simulink model "s_as_lqr"  (Simulink 8.7)
settings: Solver=ode1  StartTime=0.0  StopTime=inf  FixedStep=0.001  RelTol=1e-3
values from neighbouring files (symbols this model uses):
  A = [ 0 1 0 -1 ... (first row only)    [FitnessFunc.m]    (also in FitnessFunc_ISE.m; FitnessFunc_ITAE.m; setup_as.m)
  B = [0  0 ... (first row only)    [FitnessFunc.m]    (also in FitnessFunc_ISE.m; FitnessFunc_ITAE.m; setup_as.m = [0  0 ; 0 1/ms ; -1  0 ; bus/mu -1/mu ])
  C = [ 1 0 0 0 ... (first row only)    [FitnessFunc.m]    (also in FitnessFunc_ISE.m; FitnessFunc_ITAE.m; setup_as.m = [ 1 0 0 0 ; -ks/ms -bs/ms 0 bs/ms ])
  D = [0 0 ... (first row only)    [FitnessFunc.m]    (also in FitnessFunc_ISE.m; FitnessFunc_ITAE.m; setup_as.m = zeros(6,2); D(6,2)=1/ms)
  K = lqr( A, B(:,2), Q, R )    [setup_as.m]
libraries: simulink x8, quarc_library x1
settings Model: Creator=DCrymble  LastModifiedBy=amolki  SimulationMode=external  ExtModeTrigDuration=50000
settings SolverCC: PositivePriorityOrder=on
settings DataIOCC: SignalLoggingSaveFormat=ModelDataLogs
settings OptimizationCC: BooleanDataType=off  OptimizeBlockIOStorage=off  BufferReuse=off  GlobalBufferReuse=off  ExpressionFolding=off  ExpressionDepthLimit=2147483647  LocalBlockOutputs=off  InitFltsAndDblsToZero=on
settings DebuggingCC: SolverPrmCheckMsg=warning  FcnCallInpInsideContextMsg=UseLocalSettings  StateNameClashWarn=warning  StrictBusMsg=Warning
settings SFSimCC: SimParseCustomCode=off
settings RTWCC: SystemTargetFile=quarc_windows.tlc  TemplateMakefile=quarc_default_tmf  Description=QuaRC Win32 Target
settings STFCustomTargetCC: TargetPreCompLibLocation=C:\PROGRA~2\QUARC\lib\2012b\windows\release  GeneratePreprocessorConditionals=Disable all  CPPClassGenCompliant=on  SystemTargetFile=quarc_windows.tlc
settings GRTTargetCC: TargetPreCompLibLocation=C:\PROGRA~3\QUARC\lib\2016a\windows\release  ParMdlRefBuildCompliant=off  CompOptLevelCompliant=off  ConcurrentExecutionCompliant=off  CombineOutputUpdateFcns=off  MatFileLogging=off  GRTInterface=on  UseToolchainInfoCompliant=off  ExtMode=on  ExtModeMexFile=quarc_comm

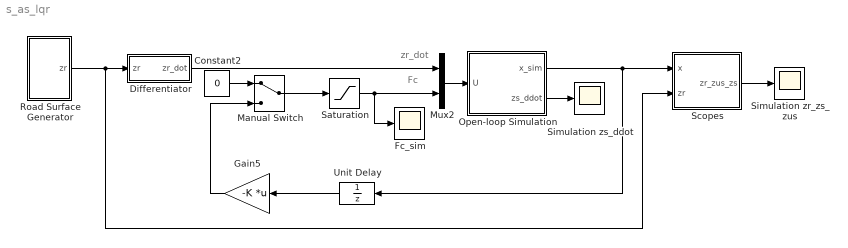
== system s_as_lqr ==
  note: zr_dot
  note: Fc
  Constant2 : Constant  Value=0
  Differentiator : Subsystem
  Fc_sim : Scope
  Gain5 : Gain  Gain=-K  Multiplication=Matrix(K*u)
  Manual Switch : ManualSwitch
  Mux2 : Mux  Inputs=2
  Open-loop Simulation : Subsystem
  Road Surface Generator : Subsystem
  Saturation : Saturate  UpperLimit=38.3  LowerLimit=-38.3
  Scopes : Subsystem
  Simulation zr_zs_zus : Scope
  Simulation zs_ddot : Scope
  Unit Delay : UnitDelay  SampleTime=-1
  wires:
  Differentiator/1(zr_dot) -> Mux2/1
  Constant2/1 -> Manual Switch/1
  Manual Switch/1 -> Saturation/1
  Mux2/1 -> Open-loop Simulation/1(U)
  Scopes/1(zr_zus_zs) -> Simulation zr_zs_zus/1
  Saturation/1 -> Mux2/2, Fc_sim/1
  Gain5/1 -> Manual Switch/2
  Open-loop Simulation/1(x_sim) -> Unit Delay/1, Scopes/1(x)
  Unit Delay/1 -> Gain5/1
  Road Surface Generator/1(zr) -> Scopes/2(zr), Differentiator/1(zr)
  Open-loop Simulation/2(zs_ddot) -> Simulation zs_ddot/1

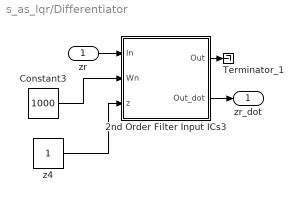
== system s_as_lqr/Differentiator ==
  zr : Inport
  2nd Order Filter Input ICs3 : Subsystem
  Constant3 : Constant  Value=1000
  Terminator_1 : Terminator
  z4 : Constant
  zr_dot : Outport
  wires:
  Constant3/1 -> 2nd Order Filter Input ICs3/2(Wn)
  z4/1 -> 2nd Order Filter Input ICs3/3(z)
  zr/1 -> 2nd Order Filter Input ICs3/1(In)
  2nd Order Filter Input ICs3/2(Out_dot) -> zr_dot/1
  2nd Order Filter Input ICs3/1(Out) -> Terminator_1/1

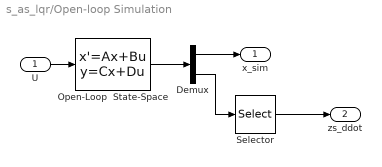
== system s_as_lqr/Open-loop Simulation ==
  U : Inport
  Demux : Demux  Outputs=[4 2]
  Open-Loop  State-Space : StateSpace  A=A  B=B  C=cat(1,eye(4), C)  D=D  X0=0
  Selector : Selector  InputPortWidth=2  IndexOptions=Index vector (dialog)  Indices=[2]  OutputSizes=1
  x_sim : Outport
  zs_ddot : Outport  Port=2
  wires:
  Open-Loop  State-Space/1 -> Demux/1
  Demux/1 -> x_sim/1
  U/1 -> Open-Loop  State-Space/1
  Demux/2 -> Selector/1
  Selector/1 -> zs_ddot/1

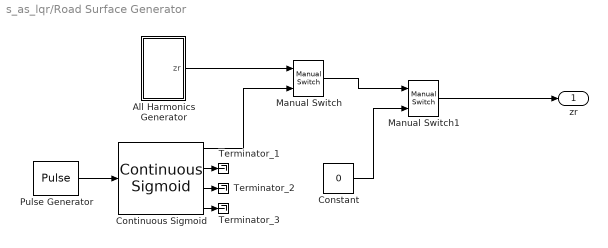
== system s_as_lqr/Road Surface Generator ==
  All Harmonics Generator : Subsystem
  Constant : Constant  Value=0
  Continuous Sigmoid : quarc_library/Sources/Sigmoids/Continuous Sigmoid  params_source=Internal (dialog parameters)  max_velocity=.6/3  max_acceleration=20  initial_position=0  initial_velocity=0  hold_off=0.5  input_sample_time=-1  output_sample_time=qc_get_step_size
  Manual Switch : simulink/Signal Routing/Manual Switch  sw=0  action=0  varsize=off
  Manual Switch1 : simulink/Signal Routing/Manual Switch  sw=1  action=0  varsize=off
  Pulse Generator : DiscretePulseGenerator  PulseType=Time based  Amplitude=0.02  Period=3  PulseWidth=50  PhaseDelay=.1
  Terminator_1 : Terminator
  Terminator_2 : Terminator
  Terminator_3 : Terminator
  zr : Outport
  wires:
  Pulse Generator/1 -> Continuous Sigmoid/1
  All Harmonics Generator/1(zr) -> Manual Switch/1
  Continuous Sigmoid/1 -> Manual Switch/2
  Constant/1 -> Manual Switch1/2
  Manual Switch/1 -> Manual Switch1/1
  Continuous Sigmoid/2 -> Terminator_1/1
  Continuous Sigmoid/3 -> Terminator_2/1
  Continuous Sigmoid/4 -> Terminator_3/1
  Manual Switch1/1 -> zr/1

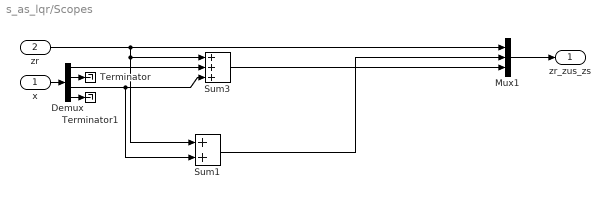
== system s_as_lqr/Scopes ==
  x : Inport
  zr : Inport  Port=2
  Demux : Demux
  Mux1 : Mux  Inputs=3
  Sum1 : Sum  Inputs=2  SaturateOnIntegerOverflow=on  InputSameDT=on  OutDataTypeStr=Inherit: Same as first input
  Sum3 : Sum  Inputs=3  SaturateOnIntegerOverflow=on  InputSameDT=on  OutDataTypeStr=Inherit: Same as first input
  Terminator : Terminator
  Terminator1 : Terminator
  zr_zus_zs : Outport
  wires:
  Demux/1 -> Sum3/2
  Demux/3 -> Sum3/3, Sum1/2
  zr/1 -> Mux1/1, Sum3/1, Sum1/1
  x/1 -> Demux/1
  Sum1/1 -> Mux1/2
  Sum3/1 -> Mux1/3
  Mux1/1 -> zr_zus_zs/1
  Demux/2 -> Terminator/1
  Demux/4 -> Terminator1/1

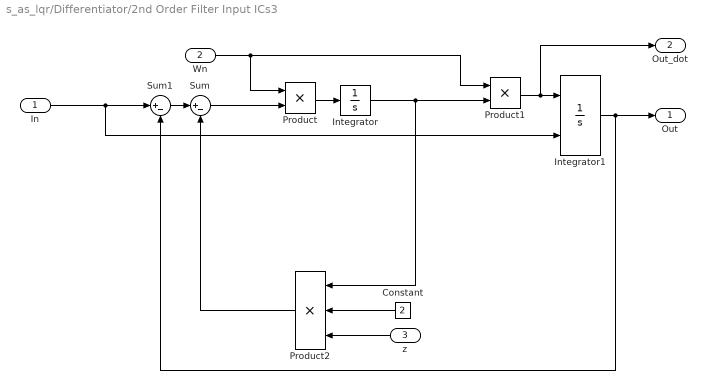
== system s_as_lqr/Differentiator/2nd Order Filter Input ICs3 ==
  In : Inport
  Wn : Inport  Port=2
  z : Inport  Port=3
  Constant : Constant  Value=2
  Integrator : Integrator
  Integrator1 : Integrator  InitialConditionSource=external
  Product : Product  RndMeth=Zero
  Product1 : Product  RndMeth=Zero
  Product2 : Product  Inputs=3  RndMeth=Zero
  Sum : Sum  Inputs=|+-
  Sum1 : Sum  Inputs=|+-
  Out : Outport
  Out_dot : Outport  Port=2
  wires:
  Constant/1 -> Product2/2
  z/1 -> Product2/3
  Product2/1 -> Sum/2
  In/1 -> Integrator1/2, Sum1/1
  Sum1/1 -> Sum/1
  Integrator1/1 -> Out/1, Sum1/2
  Integrator/1 -> Product2/1, Product1/2
  Product1/1 -> Out_dot/1, Integrator1/1
  Wn/1 -> Product1/1, Product/1
  Sum/1 -> Product/2
  Product/1 -> Integrator/1

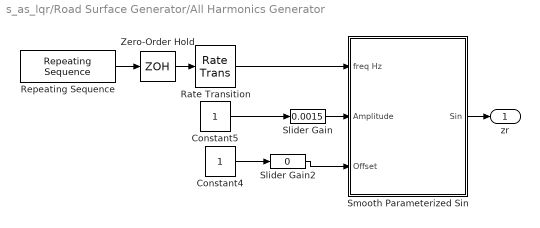
== system s_as_lqr/Road Surface Generator/All Harmonics Generator ==
  Constant4 : Constant
  Constant5 : Constant
  Rate Transition : RateTransition
  Repeating Sequence : simulink/Sources/Repeating Sequence  rep_seq_t=[0 30 30.1 ]  rep_seq_y=[1 8 1 ]
  Slider Gain : simulink/Math Operations/Slider Gain  low=0  gain=0.0015  high=0.002
  Slider Gain2 : simulink/Math Operations/Slider Gain  low=-10  gain=0  high=10
  Smooth Parameterized Sin : Subsystem  mask(Smooth Parameterized Sin Wave){}
      mask help:
      | Sin wave that will smoothly and continuously change as input
      | parameters are changed.
      |
      | Out = Amplitude * sin(freq*t) +offset
  Zero-Order Hold : ZeroOrderHold  SampleTime=.1
  zr : Outport
  wires:
  Slider Gain/1 -> Smooth Parameterized Sin/2(Amplitude)
  Slider Gain2/1 -> Smooth Parameterized Sin/3(Offset)
  Constant4/1 -> Slider Gain2/1
  Constant5/1 -> Slider Gain/1
  Repeating Sequence/1 -> Zero-Order Hold/1
  Zero-Order Hold/1 -> Rate Transition/1
  Rate Transition/1 -> Smooth Parameterized Sin/1(freq Hz)
  Smooth Parameterized Sin/1(Sin) -> zr/1

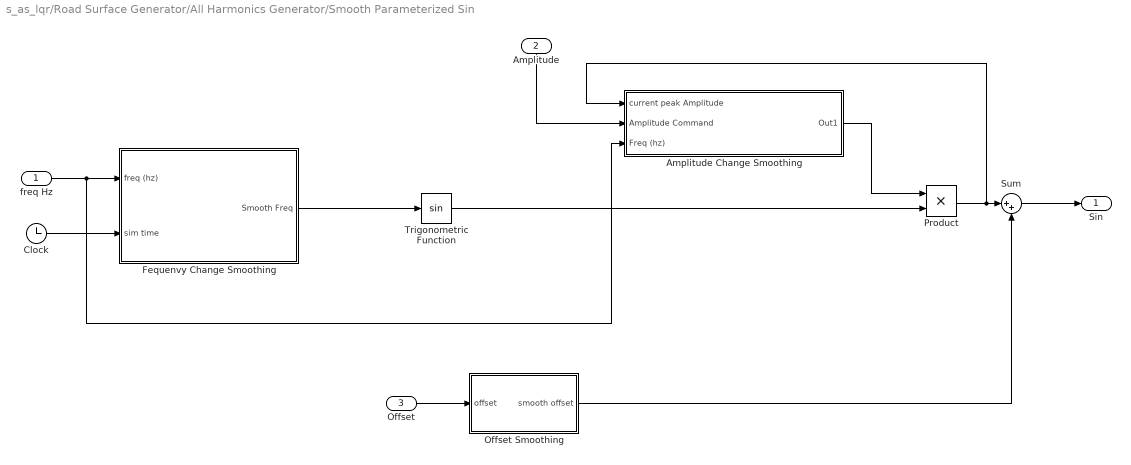
== system s_as_lqr/Road Surface Generator/All Harmonics Generator/Smooth Parameterized Sin ==
  freq Hz : Inport
  Amplitude : Inport  Port=2
  Offset : Inport  Port=3
  Amplitude Change Smoothing : Subsystem
  Clock : Clock
  Fequenvy Change Smoothing : Subsystem
  Offset Smoothing : Subsystem
  Product : Product  RndMeth=Zero
  Sum : Sum  Inputs=|++
  Trigonometric Function : Trigonometry
  Sin : Outport
  wires:
  Sum/1 -> Sin/1
  Clock/1 -> Fequenvy Change Smoothing/2(sim time)
  freq Hz/1 -> Fequenvy Change Smoothing/1(freq (hz)), Amplitude Change Smoothing/3(Freq (hz))
  Fequenvy Change Smoothing/1(Smooth Freq) -> Trigonometric Function/1
  Trigonometric Function/1 -> Product/2
  Offset Smoothing/1(smooth offset) -> Sum/2
  Offset/1 -> Offset Smoothing/1(offset)
  Product/1 -> Sum/1, Amplitude Change Smoothing/1(current peak Amplitude)
  Amplitude Change Smoothing/1(Out1) -> Product/1
  Amplitude/1 -> Amplitude Change Smoothing/2(Amplitude Command)

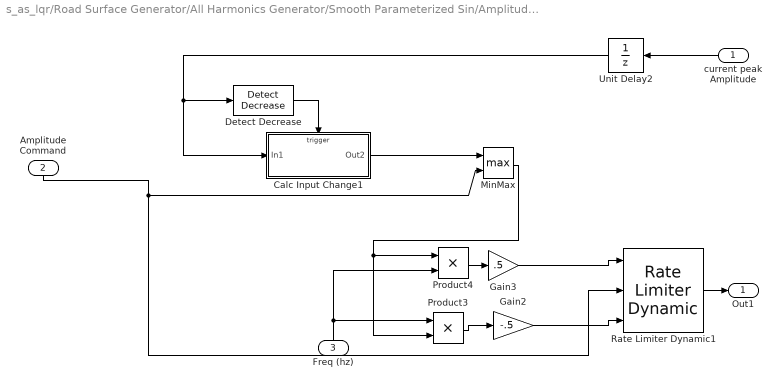
== system s_as_lqr/Road Surface Generator/All Harmonics Generator/Smooth Parameterized Sin/Amplitude Change Smoothing ==
  current peak Amplitude : Inport
  Amplitude Command : Inport  Port=2
  Freq (hz) : Inport  Port=3
  Calc Input Change1 : Subsystem  TreatAsAtomicUnit=on
  Detect Decrease : simulink/Logic and Bit Operations/Detect Decrease  vinit=0.0  InputProcessing=Inherited  OutDataTypeStr=uint8
  Gain2 : Gain  Gain=-.5
  Gain3 : Gain  Gain=.5
  MinMax : MinMax  Function=max  Inputs=2
  Product3 : Product  RndMeth=Zero
  Product4 : Product  RndMeth=Zero
  Rate Limiter Dynamic1 : simulink/Discontinuities/Rate Limiter Dynamic
  Unit Delay2 : UnitDelay  SampleTime=-1
  Out1 : Outport
  wires:
  Gain2/1 -> Rate Limiter Dynamic1/3
  Gain3/1 -> Rate Limiter Dynamic1/1
  Amplitude Command/1 -> MinMax/2, Rate Limiter Dynamic1/2
  Product3/1 -> Gain2/1
  Product4/1 -> Gain3/1
  Detect Decrease/1 -> Calc Input Change1/Trigger
  Calc Input Change1/1(Out2) -> MinMax/1
  Unit Delay2/1 -> Calc Input Change1/1(In1), Detect Decrease/1
  MinMax/1 -> Product4/1, Product3/2
  current peak Amplitude/1 -> Unit Delay2/1
  Freq (hz)/1 -> Product3/1, Product4/2
  Rate Limiter Dynamic1/1 -> Out1/1

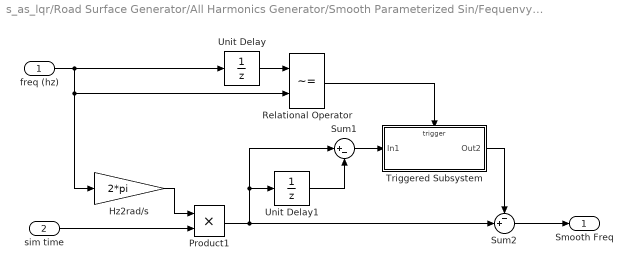
== system s_as_lqr/Road Surface Generator/All Harmonics Generator/Smooth Parameterized Sin/Fequenvy Change Smoothing ==
  freq (hz) : Inport
  sim time : Inport  Port=2
  Hz2rad/s : Gain  Gain=2*pi
  Product1 : Product  RndMeth=Zero
  Relational Operator : RelationalOperator  Operator=~=  OutDataTypeStr=boolean
  Sum1 : Sum  Inputs=|+-
  Sum2 : Sum  Inputs=-+|
  Triggered Subsystem : Subsystem  TreatAsAtomicUnit=on
  Unit Delay : UnitDelay  SampleTime=-1
  Unit Delay1 : UnitDelay  SampleTime=-1
  Smooth Freq : Outport
  wires:
  Triggered Subsystem/1(Out2) -> Sum2/1
  Unit Delay1/1 -> Sum1/2
  Relational Operator/1 -> Triggered Subsystem/Trigger
  Sum1/1 -> Triggered Subsystem/1(In1)
  Unit Delay/1 -> Relational Operator/1
  Product1/1 -> Sum2/2, Sum1/1, Unit Delay1/1
  freq (hz)/1 -> Unit Delay/1, Relational Operator/2, Hz2rad/s/1
  Sum2/1 -> Smooth Freq/1
  sim time/1 -> Product1/2
  Hz2rad/s/1 -> Product1/1

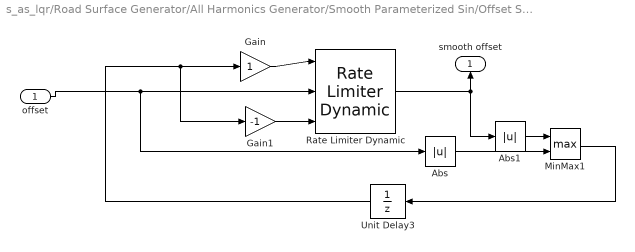
== system s_as_lqr/Road Surface Generator/All Harmonics Generator/Smooth Parameterized Sin/Offset Smoothing ==
  offset : Inport
  Abs : Abs
  Abs1 : Abs
  Gain : Gain
  Gain1 : Gain  Gain=-1
  MinMax1 : MinMax  Function=max  Inputs=2
  Rate Limiter Dynamic : simulink/Discontinuities/Rate Limiter Dynamic
  Unit Delay3 : UnitDelay  SampleTime=-1
  smooth offset : Outport
  wires:
  Rate Limiter Dynamic/1 -> Abs1/1, smooth offset/1
  offset/1 -> Rate Limiter Dynamic/2, Abs/1
  Gain1/1 -> Rate Limiter Dynamic/3
  Gain/1 -> Rate Limiter Dynamic/1
  MinMax1/1 -> Unit Delay3/1
  Unit Delay3/1 -> Gain/1, Gain1/1
  Abs/1 -> MinMax1/2
  Abs1/1 -> MinMax1/1

== system s_as_lqr/Road Surface Generator/All Harmonics Generator/Smooth Parameterized Sin/Amplitude Change Smoothing/Calc Input Change1 ==
  In1 : Inport
  Trigger : TriggerPort  VariantControl=Variant
  Out2 : Outport  InitialOutput=1000
  wires:
  In1/1 -> Out2/1

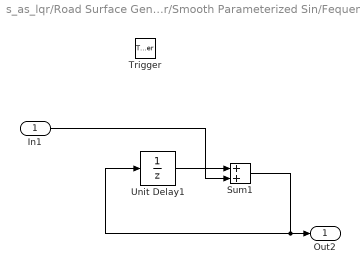
== system s_as_lqr/Road Surface Generator/All Harmonics Generator/Smooth Parameterized Sin/Fequenvy Change Smoothing/Triggered Subsystem ==
  In1 : Inport
  Trigger : TriggerPort  VariantControl=Variant
  Sum1 : Sum
  Unit Delay1 : UnitDelay  SampleTime=-1
  Out2 : Outport  InitialOutput=0
  wires:
  Unit Delay1/1 -> Sum1/1
  Sum1/1 -> Unit Delay1/1, Out2/1
  In1/1 -> Sum1/2
